simulink library "SG_library"  (R2022b)
settings: Solver=VariableStepAuto  StartTime=0.0  StopTime=10.0  RelTol=1e-3
undefined symbols (not defined in the file or in its folder): a, b, c, dfilt, GeneratorType, IO324, IO324_FPGA, IO324_src, IO334, IO334_FPGA, IO334_src, IO397, IO397_FPGA, IO397_src, repelem
libraries: speedgoatlib_hdlCoder_IO3xx x44, $bdroot x11, slrealtimeutilitieslib x9, simulink x6, hdlsllib x6, dspsrcs4 x2, dsparch4 x2
(part 3 of 3)

== system SG_library/Built elements/private/IO324_FPGA/Packer ==
  unpacked : Inport
  pack : slrealtimeutilitieslib/Bit Packing  MaskBitPatterns={[0:15 16:31 32:47 48:63 64:79 80:95 96:111 112:127 ]}  MaskPackDataType=uint32  MaskPackDataSize=4
  sSpec : SignalSpecification  OutDataTypeStr=fixdt(1,16,15)
  upconvert : DataTypeConversion  OutDataTypeStr=uint16  ConvertRealWorld=Stored Integer (SI)  SaturateOnIntegerOverflow=off
  packed : Outport
  wires:
  pack/1 -> packed/1
  upconvert/1 -> pack/1
  sSpec/1 -> upconvert/1
  unpacked/1 -> sSpec/1

== system SG_library/Built elements/private/IO324_FPGA/Packer1 ==
  unpacked : Inport
  pack : slrealtimeutilitieslib/Bit Packing  MaskBitPatterns={[0:7 8:15 ]}  MaskPackDataType=uint32  MaskPackDataSize=1
  sSpec : SignalSpecification  OutDataTypeStr=fixdt(0,8,0)
  upconvert : DataTypeConversion  OutDataTypeStr=uint8  ConvertRealWorld=Stored Integer (SI)  SaturateOnIntegerOverflow=off
  packed : Outport
  wires:
  pack/1 -> packed/1
  upconvert/1 -> pack/1
  sSpec/1 -> upconvert/1
  unpacked/1 -> sSpec/1

== system SG_library/Built elements/private/IO324_FPGA/UnPacker ==
  packed : Inport
  downconvert : DataTypeConversion  OutDataTypeStr=fixdt(1,16,15)  ConvertRealWorld=Stored Integer (SI)  SaturateOnIntegerOverflow=off
  unpack : slrealtimeutilitieslib/Bit Unpacking  SignExtend=on  MaskBitPatterns={[0:15 16:31 32:47 48:63 64:79 80:95 96:111 112:127 128:143 144:159 160:175 176:191 192:207 208:223 224:239 240:255 ]}  MaskPackDataType=uint32  MaskPackDataSize=8  MaskUnpackDataTypes={'uint16'}  MaskUnpackDataSizes={16}
  unpacked : Outport
  wires:
  downconvert/1 -> unpacked/1
  unpack/1 -> downconvert/1
  packed/1 -> unpack/1

== system SG_library/Built elements/private/IO334_FPGA/Packer ==
  unpacked : Inport
  pack : slrealtimeutilitieslib/Bit Packing  MaskBitPatterns={[0:15 16:31 32:47 48:63 64:79 80:95 96:111 112:127 128:143 144:159 160:175 176:191 192:207 208:223 224:239 240:255 ]}  MaskPackDataType=uint32  MaskPackDataSize=8
  sSpec : SignalSpecification  OutDataTypeStr=fixdt(1,16,15)
  upconvert : DataTypeConversion  OutDataTypeStr=uint16  ConvertRealWorld=Stored Integer (SI)  SaturateOnIntegerOverflow=off
  packed : Outport
  wires:
  pack/1 -> packed/1
  upconvert/1 -> pack/1
  sSpec/1 -> upconvert/1
  unpacked/1 -> sSpec/1

== system SG_library/Built elements/private/IO334_FPGA/Packer1 ==
  unpacked : Inport
  pack : slrealtimeutilitieslib/Bit Packing  MaskBitPatterns={[0:7 8:15 ]}  MaskPackDataType=uint32  MaskPackDataSize=1
  sSpec : SignalSpecification  OutDataTypeStr=fixdt(0,8,0)
  upconvert : DataTypeConversion  OutDataTypeStr=uint8  ConvertRealWorld=Stored Integer (SI)  SaturateOnIntegerOverflow=off
  packed : Outport
  wires:
  pack/1 -> packed/1
  upconvert/1 -> pack/1
  sSpec/1 -> upconvert/1
  unpacked/1 -> sSpec/1

== system SG_library/Built elements/private/IO334_FPGA/UnPacker ==
  packed : Inport
  downconvert : DataTypeConversion  OutDataTypeStr=fixdt(1,16,15)  ConvertRealWorld=Stored Integer (SI)  SaturateOnIntegerOverflow=off
  unpack : slrealtimeutilitieslib/Bit Unpacking  SignExtend=on  MaskBitPatterns={[0:15 16:31 32:47 48:63 64:79 80:95 96:111 112:127 128:143 144:159 160:175 176:191 192:207 208:223 224:239 240:255 ]}  MaskPackDataType=uint32  MaskPackDataSize=8  MaskUnpackDataTypes={'uint16'}  MaskUnpackDataSizes={16}
  unpacked : Outport
  wires:
  downconvert/1 -> unpacked/1
  unpack/1 -> downconvert/1
  packed/1 -> unpack/1

== system SG_library/Built elements/private/IO397_FPGA/Packer ==
  unpacked : Inport
  pack : slrealtimeutilitieslib/Bit Packing  MaskBitPatterns={[0:15 16:31 32:47 48:63 ]}  MaskPackDataType=uint32  MaskPackDataSize=2
  sSpec : SignalSpecification  OutDataTypeStr=fixdt(1,16,15)
  upconvert : DataTypeConversion  OutDataTypeStr=uint16  ConvertRealWorld=Stored Integer (SI)  SaturateOnIntegerOverflow=off
  packed : Outport
  wires:
  pack/1 -> packed/1
  upconvert/1 -> pack/1
  sSpec/1 -> upconvert/1
  unpacked/1 -> sSpec/1

== system SG_library/Built elements/private/IO397_FPGA/Packer1 ==
  unpacked : Inport
  pack : slrealtimeutilitieslib/Bit Packing  MaskBitPatterns={[0:7 8:15 ]}  MaskPackDataType=uint32  MaskPackDataSize=1
  sSpec : SignalSpecification  OutDataTypeStr=fixdt(0,8,0)
  upconvert : DataTypeConversion  OutDataTypeStr=uint8  ConvertRealWorld=Stored Integer (SI)  SaturateOnIntegerOverflow=off
  packed : Outport
  wires:
  pack/1 -> packed/1
  upconvert/1 -> pack/1
  sSpec/1 -> upconvert/1
  unpacked/1 -> sSpec/1

== system SG_library/Built elements/private/IO397_FPGA/UnPacker ==
  packed : Inport
  downconvert : DataTypeConversion  OutDataTypeStr=fixdt(1,16,15)  ConvertRealWorld=Stored Integer (SI)  SaturateOnIntegerOverflow=off
  unpack : slrealtimeutilitieslib/Bit Unpacking  SignExtend=on  MaskBitPatterns={[0:15 16:31 32:47 48:63 ]}  MaskPackDataType=uint32  MaskPackDataSize=2  MaskUnpackDataTypes={'uint16'}  MaskUnpackDataSizes={4}
  unpacked : Outport
  wires:
  downconvert/1 -> unpacked/1
  unpack/1 -> downconvert/1
  packed/1 -> unpack/1

== system SG_library/Source elements/Generator/gen/Switch Case Action Subsystem ==
  note: only half of the available bandwidth
  Action Port : ActionPort  InitializeStates=reset  ActionPortLabel=case [ rand_white ]:
  Discrete Filter : DiscreteFilter  Numerator=[0.5 0.5]  Denominator=[1 0.1]  a0EqualsOne=on
  random : RandomNumber  SampleTime=ts
  Out1 : Outport
  wires:
  random/1 -> Discrete Filter/1
  Discrete Filter/1 -> Out1/1

== system SG_library/Source elements/Generator/gen/Switch Case Action Subsystem1 ==
  Action Port : ActionPort  InitializeStates=reset  ActionPortLabel=case [ rand_pink ]:
  Pink Filter : DiscreteFilter  Description=https://ccrma.stanford.edu/~jos/sasp/Example_Synthesis_1_F_Noise.html  Numerator=[0.579208108 -1.113741356 0.587221367 -0.051151853]  Denominator=[1 -2.494956002 2.017265875 -0.5221894]  a0EqualsOne=on
  random : RandomNumber  SampleTime=ts
  Out1 : Outport
  wires:
  Pink Filter/1 -> Out1/1
  random/1 -> Pink Filter/1

== system SG_library/Source elements/Generator/gen/Switch Case Action Subsystem2 ==
  Action Port : ActionPort  InitializeStates=reset  ActionPortLabel=case [ sweep_lin ]:
  Gain1 : Gain  Gain=sqrt(2)
  lin_sweep : dspsrcs4/Chirp  sweep=Linear  mode=Bidirectional  f0=f0  f1=f1  t1=0.5*duration  Tsweep=0.5*duration  phase=0  Ts=ts  spf=1  datatype=Double  OutputFrames=off
  Out1 : Outport
  wires:
  lin_sweep/1 -> Gain1/1
  Gain1/1 -> Out1/1

== system SG_library/Source elements/Generator/gen/Switch Case Action Subsystem3 ==
  Action Port : ActionPort  InitializeStates=reset  ActionPortLabel=case [ sweep_log ]:
  Gain2 : Gain  Gain=sqrt(2)
  log_sweep : dspsrcs4/Chirp  sweep=Logarithmic  mode=Bidirectional  f0=f0  f1=f1  t1=0.5*duration  Tsweep=0.5*duration  phase=0  Ts=ts  spf=1  datatype=Double  OutputFrames=off
  Out1 : Outport
  wires:
  log_sweep/1 -> Gain2/1
  Gain2/1 -> Out1/1

== matlab function SG_library/Built elements/IO324_SOS/Subsystem/apply_IO_gains ==
  data: o_ao output; i_ao input; i_ctrl_limit input; i_adcGain input; i_dacGain input; o_gains output; o_ctrl_limit output
function [o_ao, o_gains, o_ctrl_limit] = fcn(i_ao, i_ctrl_limit, i_adcGain, i_dacGain)
    arguments
        i_ao            (8, 1) double
        i_ctrl_limit    (1, 1) double
        i_adcGain       (1, 1) double
        i_dacGain       (1, 1) double
    end

    switch i_dacGain
        case 1 % 10V
            adjust_dac = 0.1;
        case 2 % 5V
            adjust_dac = 0.2;
        case 3 % 2.5V
            adjust_dac = 0.4;
        otherwise
            adjust_dac = 1;
    end

    switch i_adcGain
        case 1 % 24.765V
            adjust_adc = 24.765;
        case 2 % 20.48V
            adjust_adc = 20.48;
        case 3 % 10.24
            adjust_adc = 10.24;
        case 4 % 5.12
            adjust_adc = 5.12;
        case 5 % 2.56
            adjust_adc = 2.56;
        case 6 % 1.24
            adjust_adc = 1.24;
        case 7 % 0.64
            adjust_adc = 0.64;
        otherwise
            adjust_adc = 1;
    end

    o_ao            = adjust_dac.*i_ao;
    o_gains         = adjust_dac.*adjust_adc.*[1, 1];
    o_ctrl_limit    = adjust_dac.*i_ctrl_limit;
    o_ctrl_limit(i_ctrl_limit < 0) = -1; % not considered if negative
end

== matlab function SG_library/Built elements/IO324_SOS/Subsystem1/apply_IO_gains ==
  data: o_ai output; i_ai input; i_ao_monitor input; o_ao_monitor output; i_adcGain input; i_dacGain input
function [o_ai, o_ao_monitor] = fcn(i_ai, i_ao_monitor, i_adcGain, i_dacGain)
    arguments
        i_ai            (16, 1) double
        i_ao_monitor    (1, 1) double
        i_adcGain       (1, 1) double
        i_dacGain       (1, 1) double
    end

    switch i_dacGain
        case 1 % 10V
            adjust_dac = 10;
        case 2 % 5V
            adjust_dac = 5;
        case 3 % 2.5V
            adjust_dac = 2.5;
        otherwise
            adjust_dac = 1;
    end

    switch i_adcGain
        case 1 % 24.765V
            adjust_adc = 24.765;
        case 2 % 20.48V
            adjust_adc = 20.48;
        case 3 % 10.24
            adjust_adc = 10.24;
        case 4 % 5.12
            adjust_adc = 5.12;
        case 5 % 2.56
            adjust_adc = 2.56;
        case 6 % 1.24
            adjust_adc = 1.24;
        case 7 % 0.64
            adjust_adc = 0.64;
        otherwise
            adjust_adc = 1;
    end

    o_ai            = adjust_adc.*i_ai;
    o_ao_monitor    = adjust_dac.*i_ao_monitor;
end

== matlab function SG_library/Built elements/IO397_SOS/Subsystem1/apply_IO_gains ==
  data: o_ao output; i_ao input; i_ctrl_limit input; i_adc_range input; i_dac_span input; o_gains output; o_ctrl_limit output
function [o_ao, o_gains, o_ctrl_limit] = fcn(i_ao, i_ctrl_limit, i_adc_range, i_dac_span)
    arguments
        i_ao            (4, 1) double
        i_ctrl_limit    (1, 1) double
        i_adc_range     (4, 1) double
        i_dac_span      (1, 1) double
    end

    switch i_dac_span
        case 3 % +-5V
            adjust_dac = 0.2;
        case 4 % +-10V
            adjust_dac = 0.1;
        otherwise
            error('Unsupported DAC range');
    end

    adjust_adc = ones(size(i_adc_range));
    for i = 1:numel(i_adc_range)
        switch i_adc_range(i)
            case 2 % +-5
                adjust_adc(i) = 5;
            case 3 % +-5.12
                adjust_adc(i) = 5.12;
            case 6 % +-10
                adjust_adc(i) = 10;
            case 7 % +-10.24
                adjust_adc(i) = 10.24;
            otherwise
                error('Unsupported ADC range');
        end
    end
 
    o_ao            = adjust_dac.*i_ao;
    o_gains         = adjust_dac.*adjust_adc(1:2).*[1; 1];
    o_ctrl_limit    = adjust_dac.*i_ctrl_limit;
    o_ctrl_limit(i_ctrl_limit < 0) = -1; % not considered if negative
end

== matlab function SG_library/Built elements/IO334_SOS/Subsystem/get_adc_ticks ==
  data: i_ts input; i_adc_ticks output; i_ts_default input
function i_adc_ticks = fcn(i_ts, i_ts_default)
    arguments
        i_ts (1, 1) double
        i_ts_default (1, 1) double
    end
    F_FPGA = 1e8; % FPGA frequency
    if i_ts == -1
        i_adc_ticks = uint32(F_FPGA*i_ts_default);
    else
        i_adc_ticks = uint32(F_FPGA*i_ts);
    end
end

== matlab function SG_library/Built elements/IO334_SOS/Subsystem/get_csr ==
  data: i_rst input; o_csr output; i_ctrl_on input
function o_csr = fnc(i_rst, i_ctrl_on)
    arguments
        i_rst (1, 1) logical
        i_ctrl_on (1, 1) logical
    end

    o_csr = uint8(0);
    o_csr = bitset(o_csr, 1, i_rst);
    o_csr = bitset(o_csr, 2, i_ctrl_on);
end

== matlab function SG_library/Built elements/IO334_SOS/Subsystem1/apply_IO_gains ==
  data: o_ai output; i_ai input; i_ao_monitor input; o_ao_monitor output; i_dac_span input
function [o_ai, o_ao_monitor] = fcn(i_ai, i_ao_monitor, i_dac_span)
    arguments
        i_ai            (16, 1) double
        i_ao_monitor    (1, 1) double
        i_dac_span      (1, 1) double
    end

    adjust_adc = 20; % 20V FS because of true differential (+-10 per CH)

    switch i_dac_span
        case {1, 2} % +-10V
            adjust_dac = 10;
        case 3 % +-5V
            adjust_dac = 5;
        case 4 % +-2.5V
            adjust_dac = 2.5;
        otherwise
            adjust_dac = 1;
    end

    o_ai            = adjust_adc.*i_ai;
    o_ao_monitor    = adjust_dac.*i_ao_monitor;
end

== matlab function SG_library/Built elements/IO397_SOS/Subsystem1/get_csr ==
  data: i_rst input; o_csr output; i_ctrl_on input
function o_csr = fnc(i_rst, i_ctrl_on)
    arguments
        i_rst (1, 1) logical
        i_ctrl_on (1, 1) logical
    end

    o_csr = uint8(0);
    o_csr = bitset(o_csr, 1, i_rst);
    o_csr = bitset(o_csr, 2, i_ctrl_on);
end

== matlab function SG_library/Built elements/IO397_SOS/Subsystem/MATLAB Function ==
  data: i_monitor input size=1; o_monitor output size=1; i_ai input size=4; o_ai output size=4; i_range input size=4; i_span input size=1
function [o_monitor, o_ai] = fnc(i_monitor, i_ai, i_range, i_span)
    arguments
        i_monitor   (1, 1) double
        i_ai        (4, 1) double
        i_range     (4, 1) double
        i_span      (1, 1) double
    end

    switch i_span
        case 3 % -5 to 5
            adjust_dac = 5;
        case 4 % -10 to 10
            adjust_dac = 10;
        otherwise
            error('Unsupported DAC range');
    end

    adjust_adc = ones(size(i_range));
    for i = 1:numel(i_range)
        switch i_range(i)
            case 2 % -5 to 5
                adjust_adc(i) = 5;
            case 3 % -5.12 to 5.12
                adjust_adc(i) = 5.12;
            case 6 % -10 to 10
                adjust_adc(i) = 10;
            case 7 % -10.24 to 10.24
                adjust_adc(i) = 10.24;
            otherwise
                error('Unsupported ADC range');
        end
    end

    o_monitor = adjust_dac.*i_monitor;
    o_ai = adjust_adc.*i_ai;
end

== matlab function SG_library/Source elements/Generator/gen/MATLAB Function ==
  data: u input; y output; t input
function y = fcn(u, t)
    t = 2*t;
    if t < 1
        y = u*t;
    else
        y = u;
    end
end

== matlab function SG_library/Built elements/IO397_SOS/Subsystem1/get_adc_ticks ==
  data: i_ts input; i_adc_ticks output; i_ts_default input
function i_adc_ticks = fcn(i_ts, i_ts_default)
    arguments
        i_ts (1, 1) double
        i_ts_default (1, 1) double
    end
    F_FPGA = 1e8; % FPGA frequency
    if i_ts == -1
        i_adc_ticks = uint32(F_FPGA*i_ts_default);
    else
        i_adc_ticks = uint32(F_FPGA*i_ts);
    end
end

== matlab function SG_library/Built elements/IO334_SOS/Subsystem/apply_IO_gains ==
  data: o_ao output; i_ao input; i_ctrl_limit input; i_dac_range input; o_gains output; o_ctrl_limit output
function [o_ao, o_gains, o_ctrl_limit] = fcn(i_ao, i_ctrl_limit, i_dac_range)
    arguments
        i_ao            (16, 1) double
        i_ctrl_limit    (1, 1) double
        i_dac_range     (1, 1) double
    end

    adjust_adc = 20; % 20V FS because of true differential (+-10 per CH)

    switch i_dac_range
        case {1,2} % +-10V
            adjust_dac = 0.1;
        case 3 % +-5V
            adjust_dac = 0.2;
        case 4 % +-2.5V
            adjust_dac = 0.4;
        otherwise
            adjust_dac = 1;
    end

    o_ao            = adjust_dac.*i_ao;
    o_gains         = adjust_dac.*adjust_adc.*[1, 1];
    o_ctrl_limit    = adjust_dac.*i_ctrl_limit;
    o_ctrl_limit(i_ctrl_limit < 0) = -1; % not considered if negative
end

== matlab function SG_library/Source elements/Discrete SOS section DFI serial/MATLAB Function ==
  data: cntr input; a output; u0 input; u1 input; u2 input; y1 input; y2 input; sos input; idx input; fb input; b output; c output
function [a, b, c] = serializer(cntr, u0, u1, u2, y1, y2, sos, idx, fb)
    N = width(sos)/6;

    switch cntr
        case 0
            a = u0;
            b = sos(:, idx);
            c = zeros(size(fb), 'like', fb);
        case 1
            a = u1;
            b = sos(:, idx + N);
            c = fb;
        case 2
            a = u2;
            b = sos(:, idx + 2*N);
            c = fb;
        case 3
            a = y1;
            b = -sos(:, idx + 4*N);
            c = fb;
        otherwise
            a = y2;
            b = -sos(:, idx + 5*N);
            c = fb;
    end
end

== matlab function SG_library/Built elements/IO324_SOS/Subsystem/get_csr ==
  data: i_rst input; o_csr output; i_ctrl_on input
function o_csr = fnc(i_rst, i_ctrl_on)
    arguments
        i_rst (1, 1) logical
        i_ctrl_on (1, 1) logical
    end

    o_csr = uint8(0);
    o_csr = bitset(o_csr, 1, i_rst);
    o_csr = bitset(o_csr, 2, i_ctrl_on);
end

== matlab function SG_library/Built elements/IO324_SOS/Subsystem/get_adc_ticks ==
  data: i_ts input; i_adc_ticks output; i_ts_default input
function i_adc_ticks = fcn(i_ts, i_ts_default)
    arguments
        i_ts (1, 1) double
        i_ts_default (1, 1) double
    end
    F_FPGA = 1e8; % FPGA frequency
    if i_ts == -1
        i_adc_ticks = uint32(F_FPGA*i_ts_default);
    else
        i_adc_ticks = uint32(F_FPGA*i_ts);
    end
end
